simulink model "VariableCapacitor"  (R2017a)
settings: Solver=VariableStepAuto  StartTime=0.0  StopTime=0.2  MaxStep=1e-4  RelTol=1e-3
libraries: powerlib x9
settings Model: Creator=Ugur  LastModifiedBy=Ugur

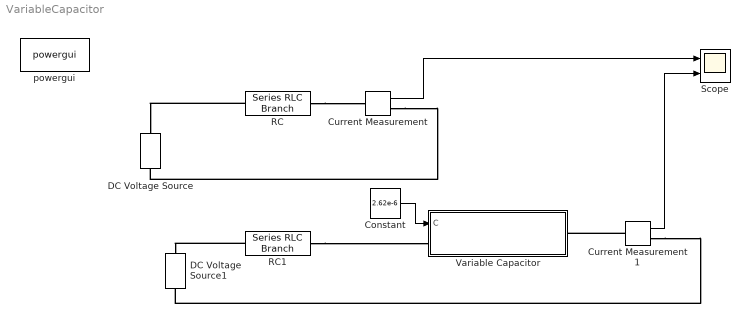
== system VariableCapacitor ==
  Constant : Constant  Value=2.62e-6  VectorParams1D=off
  Current Measurement : powerlib/Measurements/Current Measurement  PhasorSimulation=off  OutputType=Complex  PSBequivalent=0
  Current Measurement1 : powerlib/Measurements/Current Measurement  PhasorSimulation=off  OutputType=Complex  PSBequivalent=0
  DC Voltage Source : powerlib/Electrical Sources/DC Voltage Source  Amplitude=100  Measurements=None
  DC Voltage Source1 : powerlib/Electrical Sources/DC Voltage Source  Amplitude=100  Measurements=None
  RC : powerlib/Elements/Series RLC Branch  LConnTagsString=__new0  RConnTagsString=__new0  BranchType=RLC  Resistance=1.27  Inductance=107.42e-3  SetiL0=off  InitialCurrent=0  Capacitance=2.62e-6  Setx0=on  InitialVoltage=0  Measurements=None
  RC1 : powerlib/Elements/Series RLC Branch  LConnTagsString=__new0  RConnTagsString=__new0  BranchType=RL  Resistance=1.27  Inductance=107.42e-3  SetiL0=off  InitialCurrent=0  Capacitance=2.62e-6  Setx0=off  InitialVoltage=0  Measurements=None
  Scope : Scope  NumInputPorts=2
  Variable Capacitor : Subsystem  mask{Vinit=0, Cinit=2.62e-6}
      mask prompts: Vinit "Initial capacitor voltage (V)"; Cinit "Initial capacitance (F)"
      mask help: Note: capacitor voltage initialization is performed for DC only.
      mask Display: disp('Variable Capacitor')
  powergui : powerlib/powergui  SimulationMode=Continuous  SampleTime=0  frequency=60  Iterations=50  frequencyindice=0  Pbase=100e6  ErrMax=1e-4  UnitsV=kV  UnitsW=MW  buscounter=0  FunctionMessages=off  echomessages=off  EnableUseOfTLC=off  CurrentSourceSwitches=off  DisableSnubberDevices=off  DisableRonSwitches=off  DisableVfSwitches=off  DisplayEquations=off  SolverType=Tustin/Backward Euler (TBE)  Interpol=off  ExternalGateDelay=off  methode=off  Ts=100  x0status=zero  SPID=on  SwTol=0  HookPort=off  RestoreLinks=warning  ResistiveCurrentMeasurement=off  Frange=[0:2:500]  Ylog=off  Xlog=on  ShowGrid=off  save=off  variable=ZData  structure=0  ZoomFFT=on  StartTime=0.0  cycles=1  DisplayStyle=1  fundamental=60  FreqAxis=off  MaxFrequency=1000  frequencyindicesteady=60  RmsSteady=1  display=off
  wires:
  Current Measurement/1 -> Scope/1
  Current Measurement1/1 -> Scope/2
  Constant/1 -> Variable Capacitor/1(C)
  connections:
  RC/LConn1 -- DC Voltage Source/RConn1
  RC/RConn1 -- Current Measurement/LConn1
  Current Measurement/RConn1 -- DC Voltage Source/LConn1
  RC1/LConn1 -- DC Voltage Source1/RConn1
  Current Measurement1/LConn1 -- Variable Capacitor/RConn1
  Current Measurement1/RConn1 -- DC Voltage Source1/LConn1
  RC1/RConn1 -- Variable Capacitor/LConn1

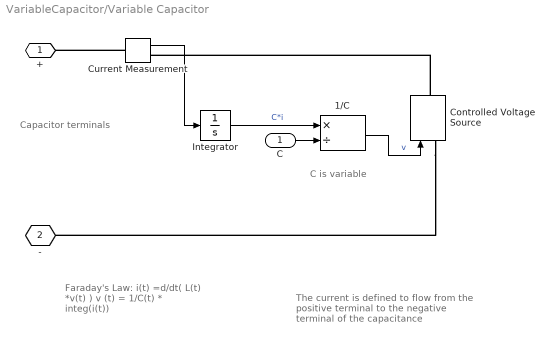
== system VariableCapacitor/Variable Capacitor ==
  note: C is variable
  note: Capacitor
      | terminals
  note: The current is defined to flow from
      |  the positive terminal to the negative
      | terminal of the capacitance
  note: Faraday's Law:
      |
      | i(t) =d/dt( L(t) *v(t) )
      | v (t) = 1/C(t) * integ(i(t))
  C : Inport
  1/C : Product  Inputs=*/  SaturateOnIntegerOverflow=on  OutDataTypeStr=Inherit: Same as first input
  Controlled Voltage Source : powerlib/Electrical Sources/Controlled Voltage Source  Initialize=on  Source_Type=DC  Amplitude=0  Phase=0  Frequency=0  Measurements=None
  Current Measurement : powerlib/Measurements/Current Measurement  PhasorSimulation=off  OutputType=Complex  PSBequivalent=0
  Integrator : Integrator  InitialCondition=Cinit*Vinit
  + : PMIOPort  Port=1  Side=Left
  - : PMIOPort  Port=2  Side=Right
  wires:
  C/1 -> 1/C/2
  Integrator/1 -> 1/C/1  "C*i"
  Current Measurement/1 -> Integrator/1
  1/C/1 -> Controlled Voltage Source/1  "v"
  connections:
  Current Measurement/LConn1 -- +/RConn1
  Controlled Voltage Source/RConn1 -- Current Measurement/RConn1
  Controlled Voltage Source/LConn1 -- -/RConn1
